simulink model "h2s"  (Simulink 7.9)
settings: Solver=ode3  StartTime=0.0  StopTime=15.0  FixedStep=0.0001  RelTol=1e-3
settings Model: Creator=touch_sky_  LastModifiedBy=mingshuai

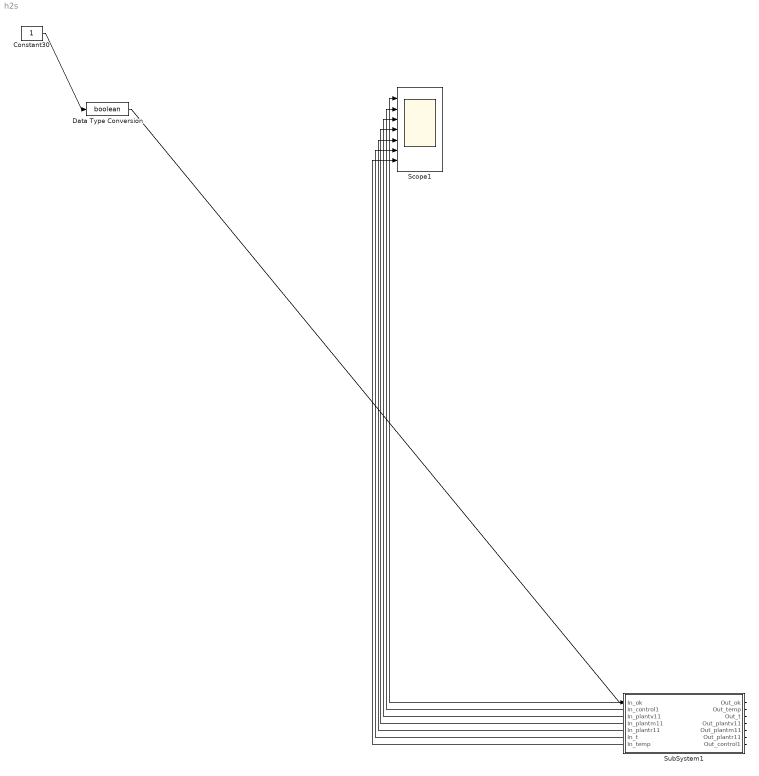
== system h2s ==
  Constant30 : Constant
  Data Type Conversion : DataTypeConversion  OutDataTypeStr=boolean
  Scope1 : Scope  NumInputPorts=7
      settings: YMin=-5~-5~-5~-5~-5~-5~-5  YMax=5~5~5~5~5~5~5  MaxDataPoints=500000
  SubSystem1 : Subsystem
  wires:
  Constant30/1 -> Data Type Conversion/1
  Data Type Conversion/1 -> SubSystem1/1(In_ok)
  SubSystem1/1(Out_ok) -> Scope1/1
  SubSystem1/2(Out_temp) -> Scope1/2
  SubSystem1/3(Out_t) -> Scope1/3
  SubSystem1/4(Out_plantv11) -> Scope1/4
  SubSystem1/5(Out_plantm11) -> Scope1/5
  SubSystem1/6(Out_plantr11) -> Scope1/6
  SubSystem1/7(Out_control1) -> Scope1/7

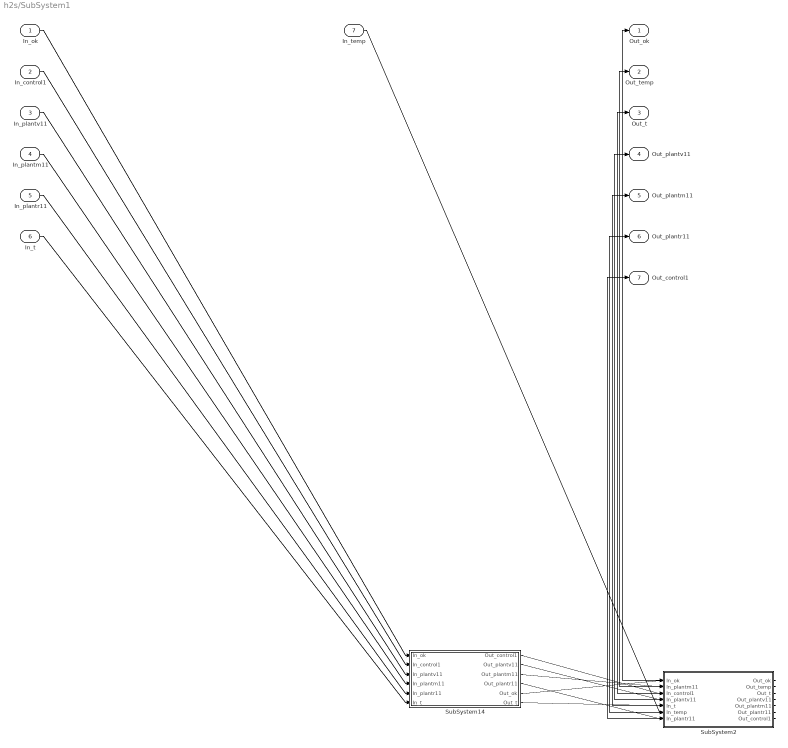
== system h2s/SubSystem1 ==
  In_ok : Inport
  In_control1 : Inport  Port=2
  In_plantv11 : Inport  Port=3
  In_plantm11 : Inport  Port=4
  In_plantr11 : Inport  Port=5
  In_t : Inport  Port=6
  In_temp : Inport  Port=7
  SubSystem14 : Subsystem
  SubSystem2 : Subsystem
  Out_ok : Outport
  Out_temp : Outport  Port=2
  Out_t : Outport  Port=3
  Out_plantv11 : Outport  Port=4
  Out_plantm11 : Outport  Port=5
  Out_plantr11 : Outport  Port=6
  Out_control1 : Outport  Port=7
  wires:
  In_ok/1 -> SubSystem14/1(In_ok)
  In_control1/1 -> SubSystem14/2(In_control1)
  In_plantv11/1 -> SubSystem14/3(In_plantv11)
  In_plantm11/1 -> SubSystem14/4(In_plantm11)
  In_plantr11/1 -> SubSystem14/5(In_plantr11)
  In_t/1 -> SubSystem14/6(In_t)
  SubSystem14/5(Out_ok) -> SubSystem2/1(In_ok)
  SubSystem14/3(Out_plantm11) -> SubSystem2/2(In_plantm11)
  SubSystem14/1(Out_control1) -> SubSystem2/3(In_control1)
  SubSystem14/2(Out_plantv11) -> SubSystem2/4(In_plantv11)
  SubSystem14/6(Out_t) -> SubSystem2/5(In_t)
  In_temp/1 -> SubSystem2/6(In_temp)
  SubSystem14/4(Out_plantr11) -> SubSystem2/7(In_plantr11)
  SubSystem2/1(Out_ok) -> Out_ok/1
  SubSystem2/2(Out_temp) -> Out_temp/1
  SubSystem2/3(Out_t) -> Out_t/1
  SubSystem2/4(Out_plantv11) -> Out_plantv11/1
  SubSystem2/5(Out_plantm11) -> Out_plantm11/1
  SubSystem2/6(Out_plantr11) -> Out_plantr11/1
  SubSystem2/7(Out_control1) -> Out_control1/1

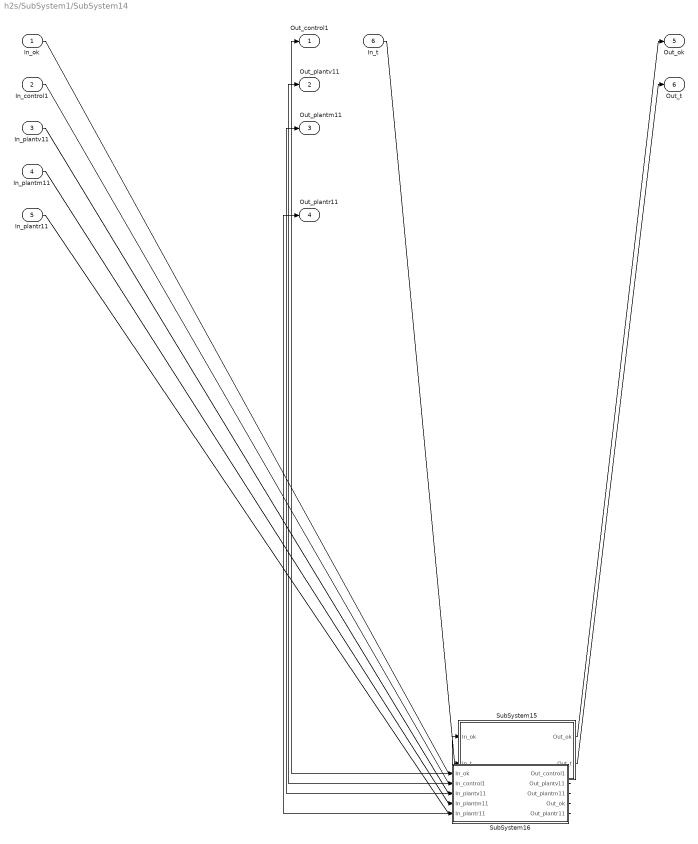
== system h2s/SubSystem1/SubSystem14 ==
  In_ok : Inport
  In_control1 : Inport  Port=2
  In_plantv11 : Inport  Port=3
  In_plantm11 : Inport  Port=4
  In_plantr11 : Inport  Port=5
  In_t : Inport  Port=6
  SubSystem15 : Subsystem
  SubSystem16 : Subsystem
  Out_control1 : Outport
  Out_plantv11 : Outport  Port=2
  Out_plantm11 : Outport  Port=3
  Out_plantr11 : Outport  Port=4
  Out_ok : Outport  Port=5
  Out_t : Outport  Port=6
  wires:
  In_ok/1 -> SubSystem16/1(In_ok)
  In_control1/1 -> SubSystem16/2(In_control1)
  In_plantv11/1 -> SubSystem16/3(In_plantv11)
  In_plantm11/1 -> SubSystem16/4(In_plantm11)
  In_plantr11/1 -> SubSystem16/5(In_plantr11)
  SubSystem16/4(Out_ok) -> SubSystem15/1(In_ok)
  In_t/1 -> SubSystem15/2(In_t)
  SubSystem16/1(Out_control1) -> Out_control1/1
  SubSystem16/2(Out_plantv11) -> Out_plantv11/1
  SubSystem16/3(Out_plantm11) -> Out_plantm11/1
  SubSystem16/5(Out_plantr11) -> Out_plantr11/1
  SubSystem15/1(Out_ok) -> Out_ok/1
  SubSystem15/2(Out_t) -> Out_t/1

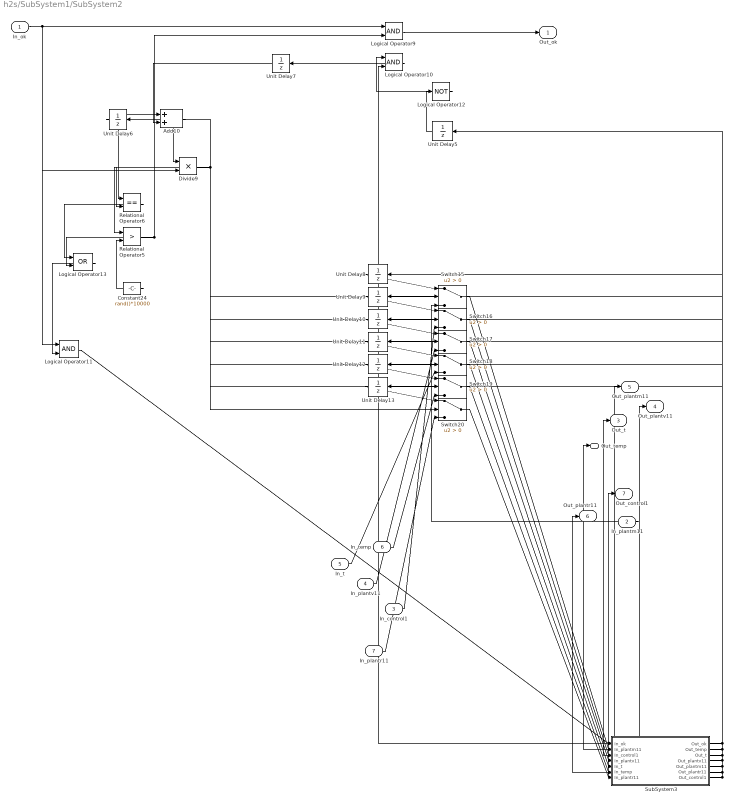
== system h2s/SubSystem1/SubSystem2 ==
  In_ok : Inport
  In_plantm11 : Inport  Port=2
  In_control1 : Inport  Port=3
  In_plantv11 : Inport  Port=4
  In_t : Inport  Port=5
  In_temp : Inport  Port=6
  In_plantr11 : Inport  Port=7
  Add10 : Sum
  Constant24 : Constant  Value=rand()*10000
  Divide9 : Product  Inputs=**  RndMeth=Zero
  Logical Operator10 : Logic  OutDataTypeStr=boolean
  Logical Operator11 : Logic  OutDataTypeStr=boolean
  Logical Operator12 : Logic  Operator=NOT  OutDataTypeStr=boolean
  Logical Operator13 : Logic  Operator=OR  OutDataTypeStr=boolean
  Logical Operator9 : Logic  OutDataTypeStr=boolean
  Relational Operator5 : RelationalOperator  Operator=>  OutDataTypeStr=boolean  InputSameDT=on
  Relational Operator6 : RelationalOperator  Operator===  OutDataTypeStr=boolean  InputSameDT=on
  SubSystem3 : Subsystem
  Switch{15..20} (6 alike) : Switch  Criteria=u2 > Threshold
  Unit Delay{5..13} (9 alike) : UnitDelay  SampleTime=0
  Out_ok : Outport
  Out_temp : Outport  Port=2
  Out_t : Outport  Port=3
  Out_plantv11 : Outport  Port=4
  Out_plantm11 : Outport  Port=5
  Out_plantr11 : Outport  Port=6
  Out_control1 : Outport  Port=7
  wires:
  In_ok/1 -> Logical Operator9/1, Divide9/2, Logical Operator11/1
  Relational Operator5/1 -> Logical Operator9/2, Logical Operator13/2
  Logical Operator9/1 -> Out_ok/1
  SubSystem3/1(Out_ok) -> Unit Delay5/1, Logical Operator10/2
  Unit Delay5/1 -> Logical Operator12/1
  Logical Operator12/1 -> Logical Operator10/1
  Logical Operator10/1 -> Unit Delay7/1
  Unit Delay7/1 -> Add10/2
  Unit Delay6/1 -> Add10/1, Relational Operator6/1
  Divide9/1 -> Unit Delay6/1, Relational Operator6/2, Relational Operator5/1, Switch15/2, Switch16/2, Switch17/2, Switch18/2, Switch19/2, Switch20/2
  Add10/1 -> Divide9/1
  Relational Operator6/1 -> Logical Operator13/1
  Constant24/1 -> Relational Operator5/2
  Logical Operator13/1 -> Logical Operator11/2
  Logical Operator11/1 -> SubSystem3/1(In_ok)
  SubSystem3/2(Out_temp) -> Out_temp/1, Unit Delay12/1
  SubSystem3/3(Out_t) -> Out_t/1, Unit Delay11/1
  SubSystem3/4(Out_plantv11) -> Out_plantv11/1, Unit Delay10/1
  SubSystem3/5(Out_plantm11) -> Out_plantm11/1, Unit Delay8/1
  SubSystem3/6(Out_plantr11) -> Out_plantr11/1, Unit Delay13/1
  SubSystem3/7(Out_control1) -> Out_control1/1, Unit Delay9/1
  Unit Delay8/1 -> Switch15/1
  In_plantm11/1 -> Switch15/3
  Switch15/1 -> SubSystem3/2(In_plantm11)
  Unit Delay9/1 -> Switch16/1
  In_control1/1 -> Switch16/3
  Switch16/1 -> SubSystem3/3(In_control1)
  Unit Delay10/1 -> Switch17/1
  In_plantv11/1 -> Switch17/3
  Switch17/1 -> SubSystem3/4(In_plantv11)
  Unit Delay11/1 -> Switch18/1
  In_t/1 -> Switch18/3
  Switch18/1 -> SubSystem3/5(In_t)
  Unit Delay12/1 -> Switch19/1
  In_temp/1 -> Switch19/3
  Switch19/1 -> SubSystem3/6(In_temp)
  Unit Delay13/1 -> Switch20/1
  In_plantr11/1 -> Switch20/3
  Switch20/1 -> SubSystem3/7(In_plantr11)

== system h2s/SubSystem1/SubSystem14/SubSystem15 ==
  In_ok : Inport
  In_t : Inport  Port=2
  Constant25 : Constant  Value=0
  Switch21 : Switch  Criteria=u2 > Threshold
  Switch22 : Switch  Criteria=u2 > Threshold
  Unit Delay14 : UnitDelay  SampleTime=0
  Unit Delay15 : UnitDelay  SampleTime=0
  Out_ok : Outport
  Out_t : Outport  Port=2
  wires:
  Switch22/1 -> Out_t/1, Unit Delay15/1
  Switch21/1 -> Switch22/3
  In_ok/1 -> Unit Delay14/1, Out_ok/1, Switch21/2
  Constant25/1 -> Switch21/1
  In_t/1 -> Switch21/3
  Unit Delay15/1 -> Switch22/1
  Unit Delay14/1 -> Switch22/2

== system h2s/SubSystem1/SubSystem14/SubSystem16 ==
  In_ok : Inport
  In_control1 : Inport  Port=2
  In_plantv11 : Inport  Port=3
  In_plantm11 : Inport  Port=4
  In_plantr11 : Inport  Port=5
  SubSystem17 : Subsystem
  SubSystem18 : Subsystem
  Out_control1 : Outport
  Out_plantv11 : Outport  Port=2
  Out_plantm11 : Outport  Port=3
  Out_ok : Outport  Port=4
  Out_plantr11 : Outport  Port=5
  wires:
  In_ok/1 -> SubSystem18/1(In_ok)
  In_control1/1 -> SubSystem18/2(In_control1)
  In_plantv11/1 -> SubSystem18/3(In_plantv11)
  In_plantm11/1 -> SubSystem18/4(In_plantm11)
  SubSystem18/3(Out_ok) -> SubSystem17/1(In_ok)
  In_plantr11/1 -> SubSystem17/2(In_plantr11)
  SubSystem18/1(Out_control1) -> Out_control1/1
  SubSystem18/2(Out_plantv11) -> Out_plantv11/1
  SubSystem18/4(Out_plantm11) -> Out_plantm11/1
  SubSystem17/1(Out_ok) -> Out_ok/1
  SubSystem17/2(Out_plantr11) -> Out_plantr11/1

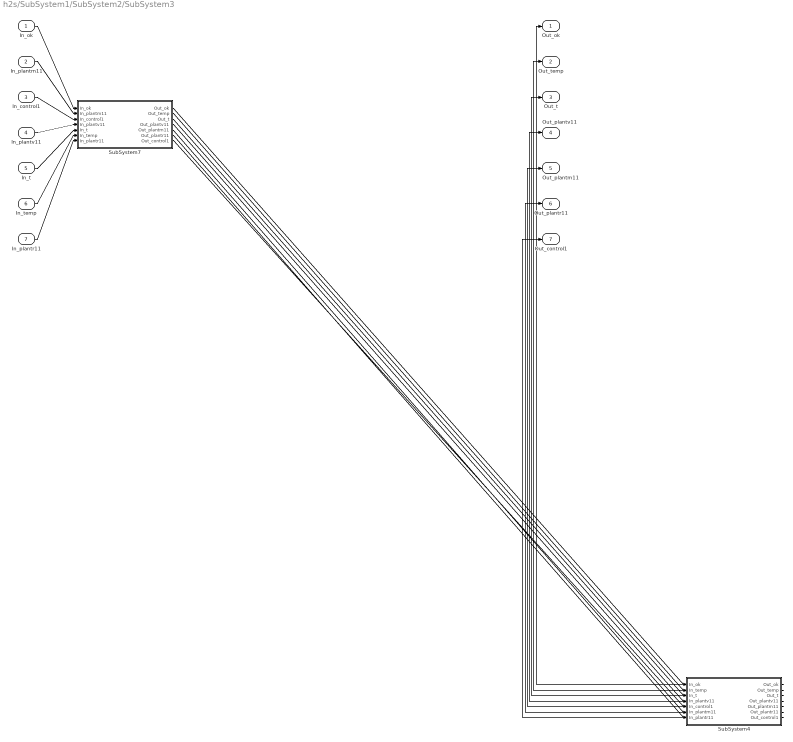
== system h2s/SubSystem1/SubSystem2/SubSystem3 ==
  In_ok : Inport
  In_plantm11 : Inport  Port=2
  In_control1 : Inport  Port=3
  In_plantv11 : Inport  Port=4
  In_t : Inport  Port=5
  In_temp : Inport  Port=6
  In_plantr11 : Inport  Port=7
  SubSystem4 : Subsystem
  SubSystem7 : Subsystem
  Out_ok : Outport
  Out_temp : Outport  Port=2
  Out_t : Outport  Port=3
  Out_plantv11 : Outport  Port=4
  Out_plantm11 : Outport  Port=5
  Out_plantr11 : Outport  Port=6
  Out_control1 : Outport  Port=7
  wires:
  In_ok/1 -> SubSystem7/1(In_ok)
  In_plantm11/1 -> SubSystem7/2(In_plantm11)
  In_control1/1 -> SubSystem7/3(In_control1)
  In_plantv11/1 -> SubSystem7/4(In_plantv11)
  In_t/1 -> SubSystem7/5(In_t)
  In_temp/1 -> SubSystem7/6(In_temp)
  In_plantr11/1 -> SubSystem7/7(In_plantr11)
  SubSystem7/1(Out_ok) -> SubSystem4/1(In_ok)
  SubSystem7/2(Out_temp) -> SubSystem4/2(In_temp)
  SubSystem7/3(Out_t) -> SubSystem4/3(In_t)
  SubSystem7/4(Out_plantv11) -> SubSystem4/4(In_plantv11)
  SubSystem7/7(Out_control1) -> SubSystem4/5(In_control1)
  SubSystem7/5(Out_plantm11) -> SubSystem4/6(In_plantm11)
  SubSystem7/6(Out_plantr11) -> SubSystem4/7(In_plantr11)
  SubSystem4/1(Out_ok) -> Out_ok/1
  SubSystem4/2(Out_temp) -> Out_temp/1
  SubSystem4/3(Out_t) -> Out_t/1
  SubSystem4/4(Out_plantv11) -> Out_plantv11/1
  SubSystem4/5(Out_plantm11) -> Out_plantm11/1
  SubSystem4/6(Out_plantr11) -> Out_plantr11/1
  SubSystem4/7(Out_control1) -> Out_control1/1

== system h2s/SubSystem1/SubSystem14/SubSystem16/SubSystem17 ==
  In_ok : Inport
  In_plantr11 : Inport  Port=2
  Constant26 : Constant  Value=30
  Switch23 : Switch  Criteria=u2 > Threshold
  Switch24 : Switch  Criteria=u2 > Threshold
  Unit Delay16 : UnitDelay  SampleTime=0
  Unit Delay17 : UnitDelay  SampleTime=0
  Out_ok : Outport
  Out_plantr11 : Outport  Port=2
  wires:
  Switch24/1 -> Out_plantr11/1, Unit Delay17/1
  Switch23/1 -> Switch24/3
  In_ok/1 -> Unit Delay16/1, Out_ok/1, Switch23/2
  Constant26/1 -> Switch23/1
  In_plantr11/1 -> Switch23/3
  Unit Delay17/1 -> Switch24/1
  Unit Delay16/1 -> Switch24/2

== system h2s/SubSystem1/SubSystem14/SubSystem16/SubSystem18 ==
  In_ok : Inport
  In_control1 : Inport  Port=2
  In_plantv11 : Inport  Port=3
  In_plantm11 : Inport  Port=4
  SubSystem19 : Subsystem
  SubSystem20 : Subsystem
  Out_control1 : Outport
  Out_plantv11 : Outport  Port=2
  Out_ok : Outport  Port=3
  Out_plantm11 : Outport  Port=4
  wires:
  In_ok/1 -> SubSystem20/1(In_ok)
  In_control1/1 -> SubSystem20/2(In_control1)
  In_plantv11/1 -> SubSystem20/3(In_plantv11)
  SubSystem20/2(Out_ok) -> SubSystem19/1(In_ok)
  In_plantm11/1 -> SubSystem19/2(In_plantm11)
  SubSystem20/1(Out_control1) -> Out_control1/1
  SubSystem20/3(Out_plantv11) -> Out_plantv11/1
  SubSystem19/1(Out_ok) -> Out_ok/1
  SubSystem19/2(Out_plantm11) -> Out_plantm11/1

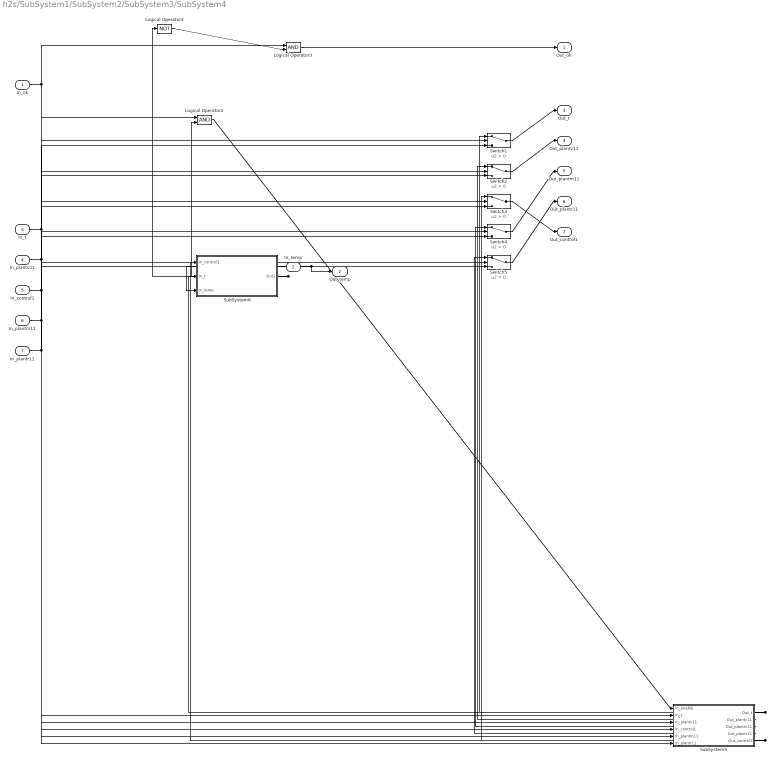
== system h2s/SubSystem1/SubSystem2/SubSystem3/SubSystem4 ==
  In_ok : Inport
  In_temp : Inport  Port=2
  In_t : Inport  Port=3
  In_plantv11 : Inport  Port=4
  In_control1 : Inport  Port=5
  In_plantm11 : Inport  Port=6
  In_plantr11 : Inport  Port=7
  Logical Operator2 : Logic  OutDataTypeStr=boolean
  Logical Operator3 : Logic  OutDataTypeStr=boolean
  Logical Operator4 : Logic  Operator=NOT  OutDataTypeStr=boolean
  SubSystem5 : Subsystem
  SubSystem6 : Subsystem
  Switch{1..5} (5 alike) : Switch  Criteria=u2 > Threshold
  Out_ok : Outport
  Out_temp : Outport  Port=2
  Out_t : Outport  Port=3
  Out_plantv11 : Outport  Port=4
  Out_plantm11 : Outport  Port=5
  Out_plantr11 : Outport  Port=6
  Out_control1 : Outport  Port=7
  wires:
  SubSystem6/1(Out1) -> Logical Operator2/2, Logical Operator4/1
  In_ok/1 -> Logical Operator2/1, Logical Operator3/1, Switch1/2, Switch2/2, Switch3/2, Switch4/2, Switch5/2
  Logical Operator2/1 -> SubSystem5/1(In_enable)
  Logical Operator4/1 -> Logical Operator3/2
  Logical Operator3/1 -> Out_ok/1
  SubSystem5/5(Out_control1) -> SubSystem6/1(In_control1), Switch3/1
  SubSystem5/1(Out_t) -> SubSystem6/2(In_t), Switch1/1
  In_temp/1 -> SubSystem6/3(In_temp), Out_temp/1
  Switch1/1 -> Out_t/1
  Switch2/1 -> Out_plantv11/1
  SubSystem5/2(Out_plantv11) -> Switch2/1
  Switch4/1 -> Out_plantm11/1
  SubSystem5/3(Out_plantm11) -> Switch4/1
  Switch3/1 -> Out_control1/1
  Switch5/1 -> Out_plantr11/1
  SubSystem5/4(Out_plantr11) -> Switch5/1
  In_t/1 -> SubSystem5/2(In_t), Switch1/3
  In_plantv11/1 -> SubSystem5/3(In_plantv11), Switch2/3
  In_control1/1 -> SubSystem5/4(In_control1), Switch3/3
  In_plantm11/1 -> SubSystem5/5(In_plantm11), Switch4/3
  In_plantr11/1 -> SubSystem5/6(In_plantr11), Switch5/3

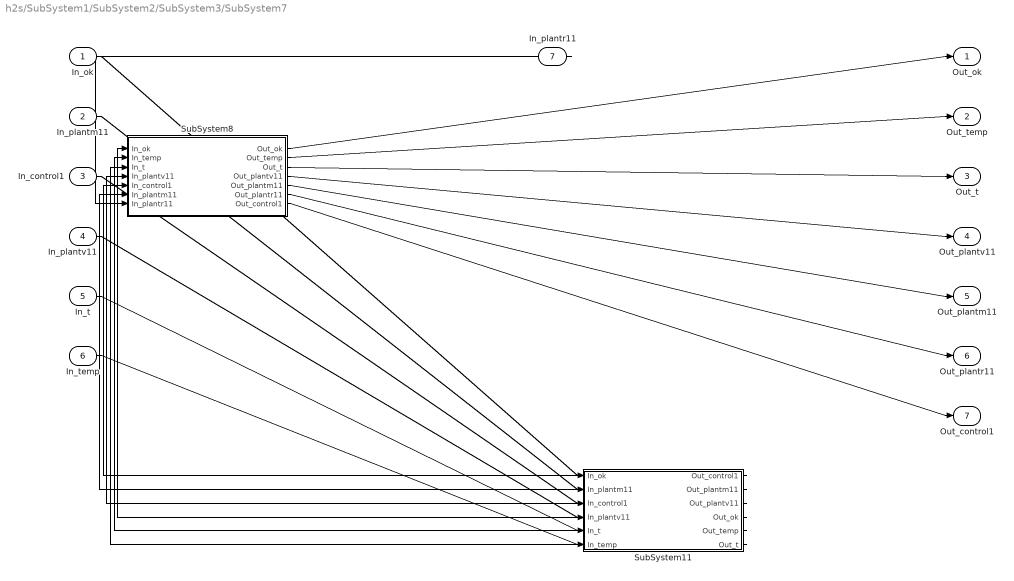
== system h2s/SubSystem1/SubSystem2/SubSystem3/SubSystem7 ==
  In_ok : Inport
  In_plantm11 : Inport  Port=2
  In_control1 : Inport  Port=3
  In_plantv11 : Inport  Port=4
  In_t : Inport  Port=5
  In_temp : Inport  Port=6
  In_plantr11 : Inport  Port=7
  SubSystem11 : Subsystem
  SubSystem8 : Subsystem
  Out_ok : Outport
  Out_temp : Outport  Port=2
  Out_t : Outport  Port=3
  Out_plantv11 : Outport  Port=4
  Out_plantm11 : Outport  Port=5
  Out_plantr11 : Outport  Port=6
  Out_control1 : Outport  Port=7
  wires:
  In_ok/1 -> SubSystem11/1(In_ok)
  In_plantm11/1 -> SubSystem11/2(In_plantm11)
  In_control1/1 -> SubSystem11/3(In_control1)
  In_plantv11/1 -> SubSystem11/4(In_plantv11)
  In_t/1 -> SubSystem11/5(In_t)
  In_temp/1 -> SubSystem11/6(In_temp)
  SubSystem11/4(Out_ok) -> SubSystem8/1(In_ok)
  SubSystem11/5(Out_temp) -> SubSystem8/2(In_temp)
  SubSystem11/6(Out_t) -> SubSystem8/3(In_t)
  SubSystem11/3(Out_plantv11) -> SubSystem8/4(In_plantv11)
  SubSystem11/1(Out_control1) -> SubSystem8/5(In_control1)
  SubSystem11/2(Out_plantm11) -> SubSystem8/6(In_plantm11)
  In_plantr11/1 -> SubSystem8/7(In_plantr11)
  SubSystem8/1(Out_ok) -> Out_ok/1
  SubSystem8/2(Out_temp) -> Out_temp/1
  SubSystem8/3(Out_t) -> Out_t/1
  SubSystem8/4(Out_plantv11) -> Out_plantv11/1
  SubSystem8/5(Out_plantm11) -> Out_plantm11/1
  SubSystem8/6(Out_plantr11) -> Out_plantr11/1
  SubSystem8/7(Out_control1) -> Out_control1/1

== system h2s/SubSystem1/SubSystem14/SubSystem16/SubSystem18/SubSystem19 ==
  In_ok : Inport
  In_plantm11 : Inport  Port=2
  Constant27 : Constant  Value=1250
  Switch25 : Switch  Criteria=u2 > Threshold
  Switch26 : Switch  Criteria=u2 > Threshold
  Unit Delay18 : UnitDelay  SampleTime=0
  Unit Delay19 : UnitDelay  SampleTime=0
  Out_ok : Outport
  Out_plantm11 : Outport  Port=2
  wires:
  Switch26/1 -> Out_plantm11/1, Unit Delay19/1
  Switch25/1 -> Switch26/3
  In_ok/1 -> Unit Delay18/1, Out_ok/1, Switch25/2
  Constant27/1 -> Switch25/1
  In_plantm11/1 -> Switch25/3
  Unit Delay19/1 -> Switch26/1
  Unit Delay18/1 -> Switch26/2

== system h2s/SubSystem1/SubSystem14/SubSystem16/SubSystem18/SubSystem20 ==
  In_ok : Inport
  In_control1 : Inport  Port=2
  In_plantv11 : Inport  Port=3
  SubSystem21 : Subsystem
  SubSystem22 : Subsystem
  Out_control1 : Outport
  Out_ok : Outport  Port=2
  Out_plantv11 : Outport  Port=3
  wires:
  In_ok/1 -> SubSystem22/1(In_ok)
  In_control1/1 -> SubSystem22/2(In_control1)
  SubSystem22/1(Out_ok) -> SubSystem21/1(In_ok)
  In_plantv11/1 -> SubSystem21/2(In_plantv11)
  SubSystem22/2(Out_control1) -> Out_control1/1
  SubSystem21/1(Out_ok) -> Out_ok/1
  SubSystem21/2(Out_plantv11) -> Out_plantv11/1

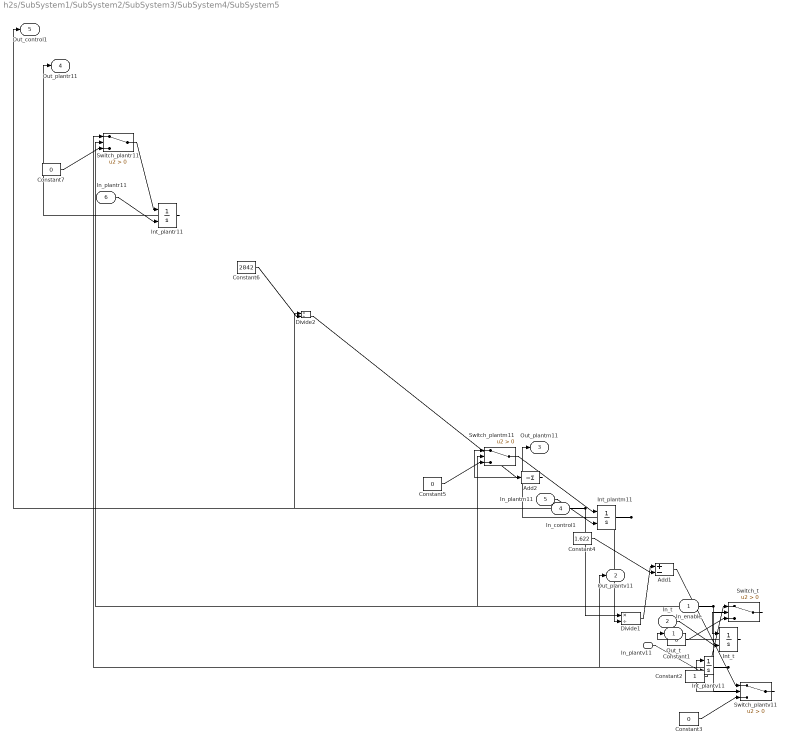
== system h2s/SubSystem1/SubSystem2/SubSystem3/SubSystem4/SubSystem5 ==
  In_enable : Inport
  In_t : Inport  Port=2
  In_plantv11 : Inport  Port=3
  In_control1 : Inport  Port=4
  In_plantm11 : Inport  Port=5
  In_plantr11 : Inport  Port=6
  Add1 : Sum  Inputs=+-
  Add2 : Sum  Inputs=-
  Constant{1,3,5,7} (4 alike) : Constant  Value=0
  Constant2 : Constant
  Constant4 : Constant  Value=1.622
  Constant6 : Constant  Value=2842
  Divide1 : Product  Inputs=*/  RndMeth=Zero
  Divide2 : Product  Inputs=*/  RndMeth=Zero
  Int_plantm11 : Integrator  InitialConditionSource=external
  Int_plantr11 : Integrator  InitialConditionSource=external
  Int_plantv11 : Integrator  InitialConditionSource=external
  Int_t : Integrator  InitialConditionSource=external
  Switch_plantm11 : Switch  Criteria=u2 > Threshold
  Switch_plantr11 : Switch  Criteria=u2 > Threshold
  Switch_plantv11 : Switch  Criteria=u2 > Threshold
  Switch_t : Switch  Criteria=u2 > Threshold
  Out_t : Outport
  Out_plantv11 : Outport  Port=2
  Out_plantm11 : Outport  Port=3
  Out_plantr11 : Outport  Port=4
  Out_control1 : Outport  Port=5
  wires:
  In_enable/1 -> Switch_t/2, Switch_plantv11/2, Switch_plantm11/2, Switch_plantr11/2
  Constant1/1 -> Switch_t/3
  Switch_t/1 -> Int_t/1
  In_t/1 -> Int_t/2
  Int_t/1 -> Out_t/1
  Constant2/1 -> Switch_t/1
  Constant3/1 -> Switch_plantv11/3
  Switch_plantv11/1 -> Int_plantv11/1
  In_plantv11/1 -> Int_plantv11/2
  Int_plantv11/1 -> Out_plantv11/1, Switch_plantr11/1
  Add1/1 -> Switch_plantv11/1
  Divide1/1 -> Add1/1
  In_control1/1 -> Divide1/1, Divide2/1, Out_control1/1
  Int_plantm11/1 -> Divide1/2, Out_plantm11/1
  Constant4/1 -> Add1/2
  Constant5/1 -> Switch_plantm11/3
  Switch_plantm11/1 -> Int_plantm11/1
  In_plantm11/1 -> Int_plantm11/2
  Add2/1 -> Switch_plantm11/1
  Divide2/1 -> Add2/1
  Constant6/1 -> Divide2/2
  Constant7/1 -> Switch_plantr11/3
  Switch_plantr11/1 -> Int_plantr11/1
  In_plantr11/1 -> Int_plantr11/2
  Int_plantr11/1 -> Out_plantr11/1

== system h2s/SubSystem1/SubSystem2/SubSystem3/SubSystem4/SubSystem6 ==
  In_control1 : Inport
  In_t : Inport  Port=2
  In_temp : Inport  Port=3
  Add3 : Sum
  Constant8 : Constant  Value=3000
  Constant9 : Constant  Value=0.128
  Logical Operator1 : Logic  OutDataTypeStr=boolean
  Relational Operator1 : RelationalOperator  Operator=<  OutDataTypeStr=boolean  InputSameDT=on
  Relational Operator2 : RelationalOperator  Operator=<  OutDataTypeStr=boolean  InputSameDT=on
  Out1 : Outport
  wires:
  Relational Operator1/1 -> Logical Operator1/1
  In_control1/1 -> Relational Operator1/1
  Constant8/1 -> Relational Operator1/2
  Relational Operator2/1 -> Logical Operator1/2
  In_t/1 -> Relational Operator2/1
  Add3/1 -> Relational Operator2/2
  In_temp/1 -> Add3/1
  Constant9/1 -> Add3/2
  Logical Operator1/1 -> Out1/1

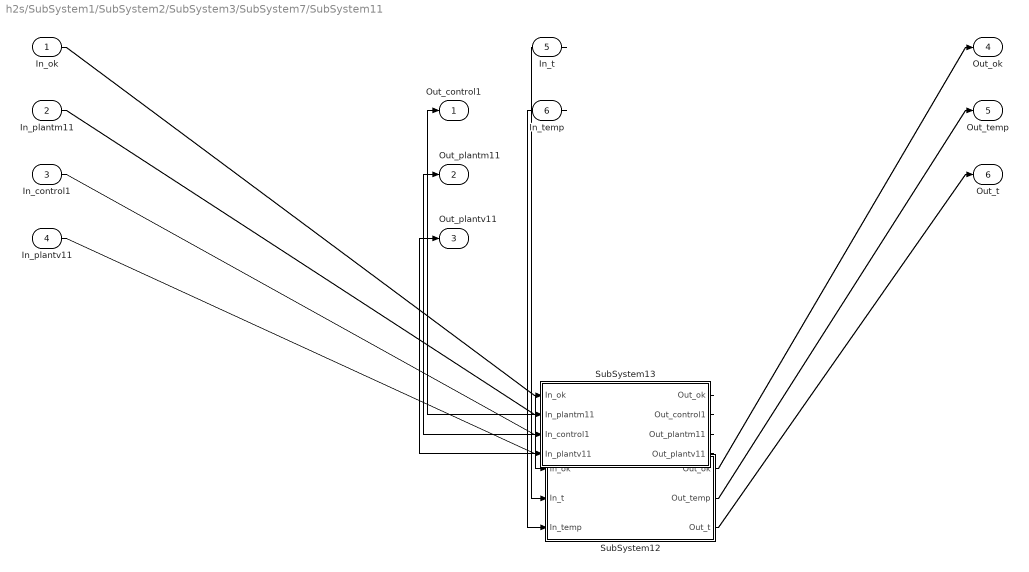
== system h2s/SubSystem1/SubSystem2/SubSystem3/SubSystem7/SubSystem11 ==
  In_ok : Inport
  In_plantm11 : Inport  Port=2
  In_control1 : Inport  Port=3
  In_plantv11 : Inport  Port=4
  In_t : Inport  Port=5
  In_temp : Inport  Port=6
  SubSystem12 : Subsystem
  SubSystem13 : Subsystem
  Out_control1 : Outport
  Out_plantm11 : Outport  Port=2
  Out_plantv11 : Outport  Port=3
  Out_ok : Outport  Port=4
  Out_temp : Outport  Port=5
  Out_t : Outport  Port=6
  wires:
  In_ok/1 -> SubSystem13/1(In_ok)
  In_plantm11/1 -> SubSystem13/2(In_plantm11)
  In_control1/1 -> SubSystem13/3(In_control1)
  In_plantv11/1 -> SubSystem13/4(In_plantv11)
  SubSystem13/1(Out_ok) -> SubSystem12/1(In_ok)
  In_t/1 -> SubSystem12/2(In_t)
  In_temp/1 -> SubSystem12/3(In_temp)
  SubSystem13/2(Out_control1) -> Out_control1/1
  SubSystem13/3(Out_plantm11) -> Out_plantm11/1
  SubSystem13/4(Out_plantv11) -> Out_plantv11/1
  SubSystem12/1(Out_ok) -> Out_ok/1
  SubSystem12/2(Out_temp) -> Out_temp/1
  SubSystem12/3(Out_t) -> Out_t/1

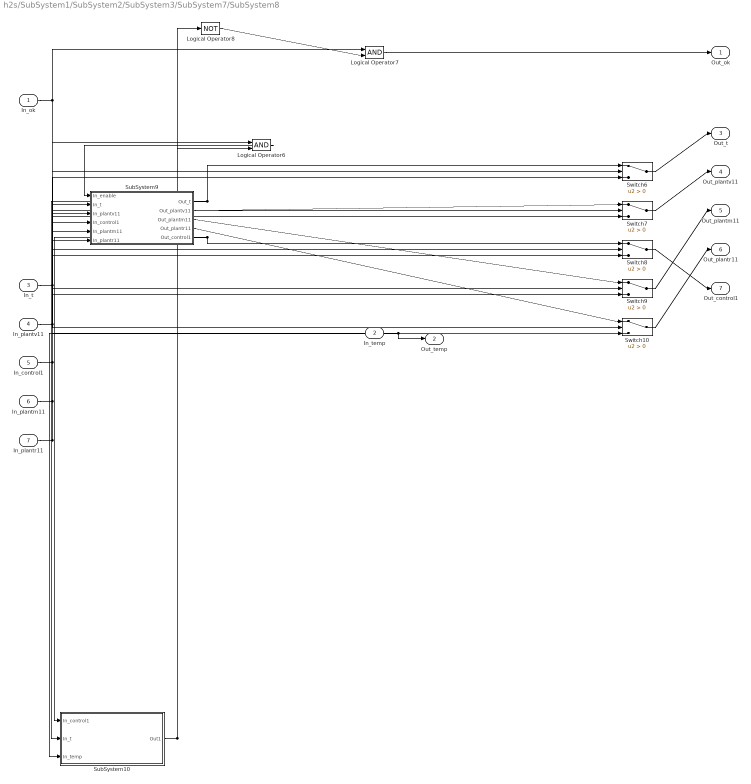
== system h2s/SubSystem1/SubSystem2/SubSystem3/SubSystem7/SubSystem8 ==
  In_ok : Inport
  In_temp : Inport  Port=2
  In_t : Inport  Port=3
  In_plantv11 : Inport  Port=4
  In_control1 : Inport  Port=5
  In_plantm11 : Inport  Port=6
  In_plantr11 : Inport  Port=7
  Logical Operator6 : Logic  OutDataTypeStr=boolean
  Logical Operator7 : Logic  OutDataTypeStr=boolean
  Logical Operator8 : Logic  Operator=NOT  OutDataTypeStr=boolean
  SubSystem10 : Subsystem
  SubSystem9 : Subsystem
  Switch{6..10} (5 alike) : Switch  Criteria=u2 > Threshold
  Out_ok : Outport
  Out_temp : Outport  Port=2
  Out_t : Outport  Port=3
  Out_plantv11 : Outport  Port=4
  Out_plantm11 : Outport  Port=5
  Out_plantr11 : Outport  Port=6
  Out_control1 : Outport  Port=7
  wires:
  SubSystem10/1(Out1) -> Logical Operator6/2, Logical Operator8/1
  In_ok/1 -> Logical Operator6/1, Logical Operator7/1, Switch6/2, Switch7/2, Switch8/2, Switch9/2, Switch10/2
  Logical Operator6/1 -> SubSystem9/1(In_enable)
  Logical Operator8/1 -> Logical Operator7/2
  Logical Operator7/1 -> Out_ok/1
  SubSystem9/5(Out_control1) -> SubSystem10/1(In_control1), Switch8/1
  SubSystem9/1(Out_t) -> SubSystem10/2(In_t), Switch6/1
  In_temp/1 -> SubSystem10/3(In_temp), Out_temp/1
  Switch6/1 -> Out_t/1
  Switch7/1 -> Out_plantv11/1
  SubSystem9/2(Out_plantv11) -> Switch7/1
  Switch9/1 -> Out_plantm11/1
  SubSystem9/3(Out_plantm11) -> Switch9/1
  Switch8/1 -> Out_control1/1
  Switch10/1 -> Out_plantr11/1
  SubSystem9/4(Out_plantr11) -> Switch10/1
  In_t/1 -> SubSystem9/2(In_t), Switch6/3
  In_plantv11/1 -> SubSystem9/3(In_plantv11), Switch7/3
  In_control1/1 -> SubSystem9/4(In_control1), Switch8/3
  In_plantm11/1 -> SubSystem9/5(In_plantm11), Switch9/3
  In_plantr11/1 -> SubSystem9/6(In_plantr11), Switch10/3

== system h2s/SubSystem1/SubSystem14/SubSystem16/SubSystem18/SubSystem20/SubSystem21 ==
  In_ok : Inport
  In_plantv11 : Inport  Port=2
  Add11 : Sum  Inputs=-
  Constant28 : Constant  Value=2
  Switch27 : Switch  Criteria=u2 > Threshold
  Switch28 : Switch  Criteria=u2 > Threshold
  Unit Delay20 : UnitDelay  SampleTime=0
  Unit Delay21 : UnitDelay  SampleTime=0
  Out_ok : Outport
  Out_plantv11 : Outport  Port=2
  wires:
  Switch28/1 -> Out_plantv11/1, Unit Delay21/1
  Switch27/1 -> Switch28/3
  In_ok/1 -> Unit Delay20/1, Out_ok/1, Switch27/2
  Add11/1 -> Switch27/1
  Constant28/1 -> Add11/1
  In_plantv11/1 -> Switch27/3
  Unit Delay21/1 -> Switch28/1
  Unit Delay20/1 -> Switch28/2

== system h2s/SubSystem1/SubSystem14/SubSystem16/SubSystem18/SubSystem20/SubSystem22 ==
  In_ok : Inport
  In_control1 : Inport  Port=2
  Constant29 : Constant  Value=2027.5
  Switch29 : Switch  Criteria=u2 > Threshold
  Switch30 : Switch  Criteria=u2 > Threshold
  Unit Delay22 : UnitDelay  SampleTime=0
  Unit Delay23 : UnitDelay  SampleTime=0
  Out_ok : Outport
  Out_control1 : Outport  Port=2
  wires:
  Switch30/1 -> Out_control1/1, Unit Delay23/1
  Switch29/1 -> Switch30/3
  In_ok/1 -> Unit Delay22/1, Out_ok/1, Switch29/2
  Constant29/1 -> Switch29/1
  In_control1/1 -> Switch29/3
  Unit Delay23/1 -> Switch30/1
  Unit Delay22/1 -> Switch30/2

== system h2s/SubSystem1/SubSystem2/SubSystem3/SubSystem7/SubSystem11/SubSystem12 ==
  In_ok : Inport
  In_t : Inport  Port=2
  In_temp : Inport  Port=3
  Switch11 : Switch  Criteria=u2 > Threshold
  Switch12 : Switch  Criteria=u2 > Threshold
  Unit Delay1 : UnitDelay  SampleTime=0
  Unit Delay2 : UnitDelay  SampleTime=0
  Out_ok : Outport
  Out_temp : Outport  Port=2
  Out_t : Outport  Port=3
  wires:
  In_ok/1 -> Unit Delay1/1, Out_ok/1, Switch11/2
  Switch12/1 -> Out_temp/1, Unit Delay2/1
  Switch11/1 -> Switch12/3
  In_t/1 -> Switch11/1, Out_t/1
  In_temp/1 -> Switch11/3
  Unit Delay2/1 -> Switch12/1
  Unit Delay1/1 -> Switch12/2

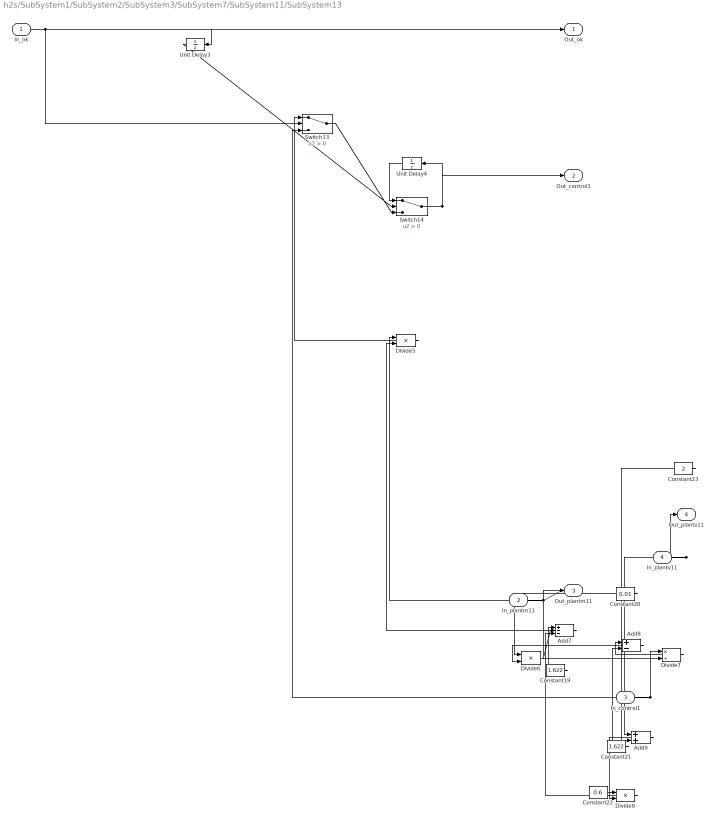
== system h2s/SubSystem1/SubSystem2/SubSystem3/SubSystem7/SubSystem11/SubSystem13 ==
  In_ok : Inport
  In_plantm11 : Inport  Port=2
  In_control1 : Inport  Port=3
  In_plantv11 : Inport  Port=4
  Add7 : Sum  Inputs=+--
  Add8 : Sum  Inputs=+-
  Add9 : Sum
  Constant19 : Constant  Value=1.622
  Constant20 : Constant  Value=0.01
  Constant21 : Constant  Value=1.622
  Constant22 : Constant  Value=0.6
  Constant23 : Constant  Value=2
  Divide5 : Product  Inputs=**  RndMeth=Zero
  Divide6 : Product  Inputs=**  RndMeth=Zero
  Divide7 : Product  Inputs=*/  RndMeth=Zero
  Divide8 : Product  Inputs=**  RndMeth=Zero
  Switch13 : Switch  Criteria=u2 > Threshold
  Switch14 : Switch  Criteria=u2 > Threshold
  Unit Delay3 : UnitDelay  SampleTime=0
  Unit Delay4 : UnitDelay  SampleTime=0
  Out_ok : Outport
  Out_control1 : Outport  Port=2
  Out_plantm11 : Outport  Port=3
  Out_plantv11 : Outport  Port=4
  wires:
  Switch14/1 -> Out_control1/1, Unit Delay4/1
  Switch13/1 -> Switch14/3
  In_ok/1 -> Unit Delay3/1, Out_ok/1, Switch13/2
  Divide5/1 -> Switch13/1
  In_plantm11/1 -> Divide5/1, Out_plantm11/1, Divide7/2
  Add7/1 -> Divide5/2
  Constant19/1 -> Add7/1
  Divide6/1 -> Add7/2
  Constant20/1 -> Divide6/1
  Add8/1 -> Divide6/2
  Divide7/1 -> Add8/1
  In_control1/1 -> Divide7/1, Switch13/3
  Constant21/1 -> Add8/2
  Divide8/1 -> Add7/3
  Constant22/1 -> Divide8/1
  Add9/1 -> Divide8/2
  In_plantv11/1 -> Out_plantv11/1, Add9/1
  Constant23/1 -> Add9/2
  Unit Delay4/1 -> Switch14/1
  Unit Delay3/1 -> Switch14/2

== system h2s/SubSystem1/SubSystem2/SubSystem3/SubSystem7/SubSystem8/SubSystem10 ==
  In_control1 : Inport
  In_t : Inport  Port=2
  In_temp : Inport  Port=3
  Add6 : Sum
  Constant17 : Constant  Value=3000
  Constant18 : Constant  Value=0.128
  Logical Operator5 : Logic  OutDataTypeStr=boolean
  Relational Operator3 : RelationalOperator  Operator=>  OutDataTypeStr=boolean  InputSameDT=on
  Relational Operator4 : RelationalOperator  Operator=<  OutDataTypeStr=boolean  InputSameDT=on
  Out1 : Outport
  wires:
  Relational Operator3/1 -> Logical Operator5/1
  In_control1/1 -> Relational Operator3/1
  Constant17/1 -> Relational Operator3/2
  Relational Operator4/1 -> Logical Operator5/2
  In_t/1 -> Relational Operator4/1
  Add6/1 -> Relational Operator4/2
  In_temp/1 -> Add6/1
  Constant18/1 -> Add6/2
  Logical Operator5/1 -> Out1/1

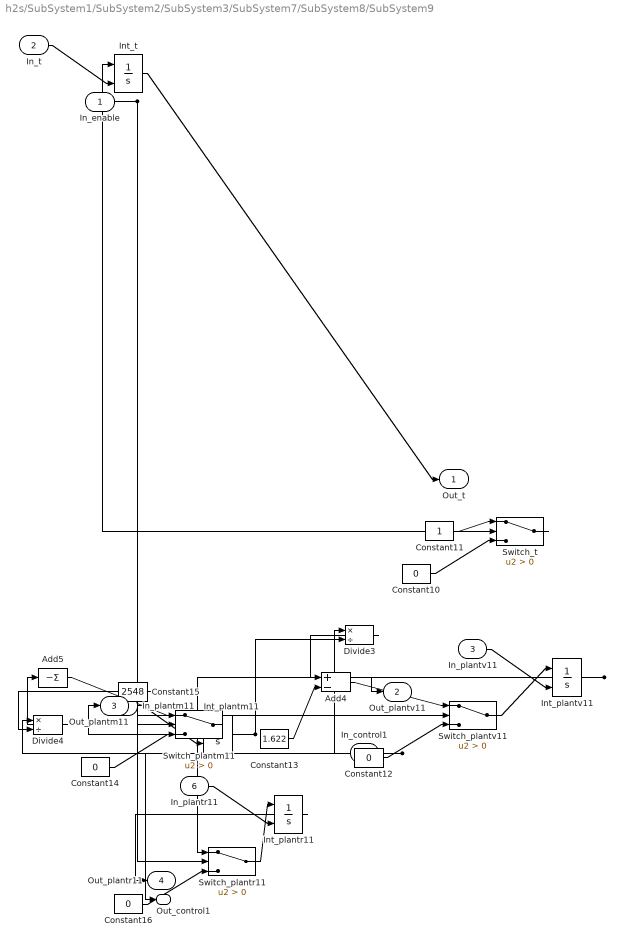
== system h2s/SubSystem1/SubSystem2/SubSystem3/SubSystem7/SubSystem8/SubSystem9 ==
  In_enable : Inport
  In_t : Inport  Port=2
  In_plantv11 : Inport  Port=3
  In_control1 : Inport  Port=4
  In_plantm11 : Inport  Port=5
  In_plantr11 : Inport  Port=6
  Add4 : Sum  Inputs=+-
  Add5 : Sum  Inputs=-
  Constant{10,12,14,16} (4 alike) : Constant  Value=0
  Constant11 : Constant
  Constant13 : Constant  Value=1.622
  Constant15 : Constant  Value=2548
  Divide3 : Product  Inputs=*/  RndMeth=Zero
  Divide4 : Product  Inputs=*/  RndMeth=Zero
  Int_plantm11 : Integrator  InitialConditionSource=external
  Int_plantr11 : Integrator  InitialConditionSource=external
  Int_plantv11 : Integrator  InitialConditionSource=external
  Int_t : Integrator  InitialConditionSource=external
  Switch_plantm11 : Switch  Criteria=u2 > Threshold
  Switch_plantr11 : Switch  Criteria=u2 > Threshold
  Switch_plantv11 : Switch  Criteria=u2 > Threshold
  Switch_t : Switch  Criteria=u2 > Threshold
  Out_t : Outport
  Out_plantv11 : Outport  Port=2
  Out_plantm11 : Outport  Port=3
  Out_plantr11 : Outport  Port=4
  Out_control1 : Outport  Port=5
  wires:
  In_enable/1 -> Switch_t/2, Switch_plantv11/2, Switch_plantm11/2, Switch_plantr11/2
  Constant10/1 -> Switch_t/3
  Switch_t/1 -> Int_t/1
  In_t/1 -> Int_t/2
  Int_t/1 -> Out_t/1
  Constant11/1 -> Switch_t/1
  Constant12/1 -> Switch_plantv11/3
  Switch_plantv11/1 -> Int_plantv11/1
  In_plantv11/1 -> Int_plantv11/2
  Int_plantv11/1 -> Out_plantv11/1, Switch_plantr11/1
  Add4/1 -> Switch_plantv11/1
  Divide3/1 -> Add4/1
  In_control1/1 -> Divide3/1, Divide4/1, Out_control1/1
  Int_plantm11/1 -> Divide3/2, Out_plantm11/1
  Constant13/1 -> Add4/2
  Constant14/1 -> Switch_plantm11/3
  Switch_plantm11/1 -> Int_plantm11/1
  In_plantm11/1 -> Int_plantm11/2
  Add5/1 -> Switch_plantm11/1
  Divide4/1 -> Add5/1
  Constant15/1 -> Divide4/2
  Constant16/1 -> Switch_plantr11/3
  Switch_plantr11/1 -> Int_plantr11/1
  In_plantr11/1 -> Int_plantr11/2
  Int_plantr11/1 -> Out_plantr11/1
